simulink model "GPCA_System_Monitor_tmp"  (Simulink 8.4)
settings: Solver=ode45  StartTime=0.0  StopTime=10.0  RelTol=1e-3
settings Model: Creator=bourbouh  LastModifiedBy=hbourbou  CovSFcnEnable=on
settings DataIOCC: LimitDataPoints=off  SaveFormat=StructureWithTime  SignalLoggingSaveFormat=Dataset
settings OptimizationCC: ExpressionDepthLimit=128
settings DebuggingCC: UnderspecifiedInitializationDetection=Simplified  MergeDetectMultiDrivingBlocksExec=error  SolverPrmCheckMsg=none  FcnCallInpInsideContextMsg=EnableAllAsError  FrameProcessingCompatibilityMsg=error  StateNameClashWarn=none
settings HardwareCC: ProdBitPerPointer=64  ProdLargestAtomicFloat=Float  ProdIntDivRoundTo=Zero  ProdEndianess=LittleEndian  ProdHWDeviceType=Specified
settings ModelReferenceCC: PropagateSignalLabelsOutOfModel=on
settings GRTTargetCC: CombineOutputUpdateFcns=on  GRTInterface=off

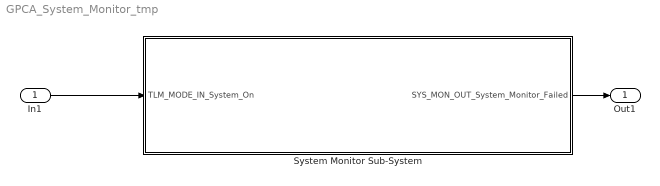
== system GPCA_System_Monitor_tmp ==
  In1 : Inport
  System Monitor Sub-System : Stateflow chart  TreatAsAtomicUnit=on
      settings: PermitHierarchicalResolution=ParametersOnly
  Out1 : Outport
  wires:
  In1/1 -> System Monitor Sub-System/1(TLM_MODE_IN_System_On)
  System Monitor Sub-System/1(SYS_MON_OUT_System_Monitor_Failed) -> Out1/1

== stateflow chart System Monitor Sub-System ==
  state System_Monitor
    entry: SYS_MON_OUT_System_Monitor_Failed=0;
    during: SYS_MON_OUT_System_Monitor_Failed=0;
    exit: SYS_MON_OUT_System_Monitor_Failed=0;
  state NOT_ON
  (default) -> System_Monitor [order 1] : [TLM_MODE_IN_System_On]
  (default) -> NOT_ON [order 2]
  NOT_ON -> System_Monitor : [TLM_MODE_IN_System_On]
  System_Monitor -> NOT_ON : [!TLM_MODE_IN_System_On]
  data: TLM_MODE_IN_System_On input boolean; SYS_MON_OUT_System_Monitor_Failed output boolean
